simulink model "van_der_Pol"  (Simulink 7.8)
settings: Solver=ode4  StartTime=0.0  StopTime=time_span  RelTol=1e-3
values from neighbouring files (symbols this model uses):
  IC = p.simulation.IC(h,i,:)    [RunVDP.m]    (also in RunVDP2.m = p.simulation.IC; RunVDP3.m = p.simulation.IC)
  outstr = model{1}    [RunVDP.m]    (also in RunVDP2.m; RunVDP3.m)
  samp_time = time_span/(p.simulation.ndata-1)    [RunVDP.m]    (also in RunVDP2.m; RunVDP3.m)
settings Model: Creator=Kourosh Danai  LastModifiedBy=BionicBill
settings DataIOCC: TimeSaveName=t  OutputSaveName=y
settings DebuggingCC: AlgebraicLoopMsg=none  FcnCallInpInsideContextMsg=Use local settings  StrictBusMsg=Warning
settings SFSimCC: SimParseCustomCode=off

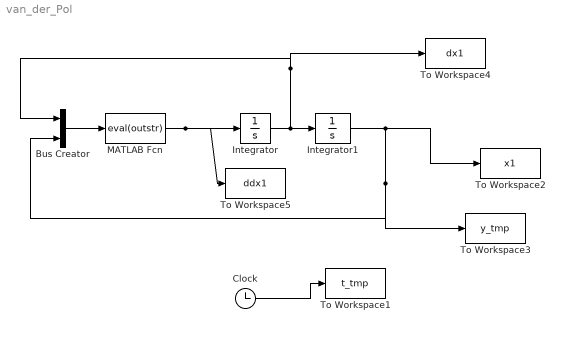
== system van_der_Pol ==
  Bus Creator : BusCreator  Inputs=2
  Clock : Clock
  Integrator : Integrator  InitialCondition=IC(1)
  Integrator1 : Integrator  InitialCondition=IC(2)
  MATLAB Fcn : MATLABFcn  MATLABFcn=eval(outstr)
  To Workspace1 : ToWorkspace  VariableName=t_tmp  SampleTime=samp_time  SaveFormat=Array
  To Workspace2 : ToWorkspace  VariableName=x1  SampleTime=samp_time  SaveFormat=Array
  To Workspace3 : ToWorkspace  VariableName=y_tmp  SampleTime=samp_time  SaveFormat=Array
  To Workspace4 : ToWorkspace  VariableName=dx1  SampleTime=samp_time  SaveFormat=Array
  To Workspace5 : ToWorkspace  VariableName=ddx1  SampleTime=samp_time  SaveFormat=Array
  wires:
  Integrator/1 -> Integrator1/1, Bus Creator/1, To Workspace4/1
  Bus Creator/1 -> MATLAB Fcn/1
  Clock/1 -> To Workspace1/1
  Integrator1/1 -> To Workspace2/1, Bus Creator/2, To Workspace3/1
  MATLAB Fcn/1 -> Integrator/1, To Workspace5/1
